simulink model "hybrid_5_bus_scan_comparison"  (R2024b)
settings: Solver=FixedStepAuto  StartTime=0  StopTime=200  FixedStep=Ts  RelTol=1e-3
PreLoadFcn:
  | Ts = 1e-5;FS_Frequency=csvread('Frequency_Sweep.csv',1,0); run lpf_param.m;
InitFcn:
  | Ts = 1e-5;FS_Frequency=csvread('Frequency_Sweep.csv',1,0); run lpf_param.m;
StartFcn:
  | Ts = 1e-5;FS_Frequency=csvread('Frequency_Sweep.csv',1,0); run lpf_param.m;
values from neighbouring files (symbols this model uses):
  D = zeros(6,4)    [TheoreticalImpedancePlot.m]    (also in TheoreticalImpedancePlotGFL.m = zeros(5,4))
  Fbase = 50    [lpf_param.m]
  fpll = 0.1    [lpf_param.m]
  k_lpf = 0.707    [lpf_param.m]
  wc_lpf = 2*pi*fc_lpf    (= 0.628318530718)    [lpf_param.m]
  x_e = [i_d; i_q; i_d_i; i_q_i; v_d_i; v_q_i; theta; v_dc; v_dc_i; i; i_i; v_lk; p_sum_i; p_lk_i]    [InterlinkAcDcB2B.m]
undefined symbols (not defined in the file or in its folder): ApparatusDiscreDamping, ApparatusPara, ApparatusPowerFlow, ApparatusType, DiscIntNeverNeededParam, OtherInputs, Wbase, Ybase, Zbase
libraries: SimplusGT x20, discretizing x12, dspindex x8, spsGroundLib x5, dspsnks4 x4, spsThreePhaseParallelRLCBranchLib x3, spsControlledVoltageSourceLib x3, spsThreePhaseSeriesRLCBranchLib x2, spsParallelRLCBranchLib x2, spsThreePhaseVIMeasurementLib x2, simulink x1, sps_lib x1
(part 1 of 2)
settings Model: Creator=gzhan  LastModifiedBy=gzhan

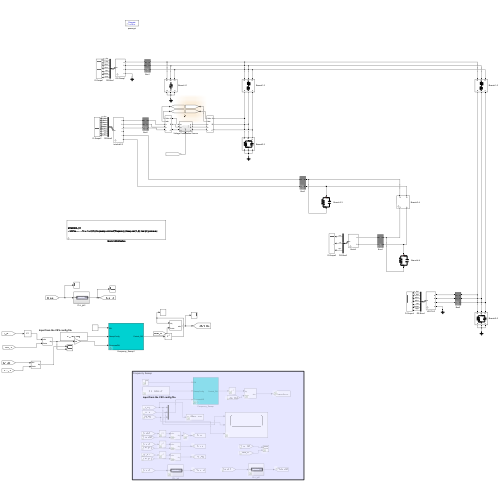
[thumbnail: Simulink's stored preview of the top-level diagram]
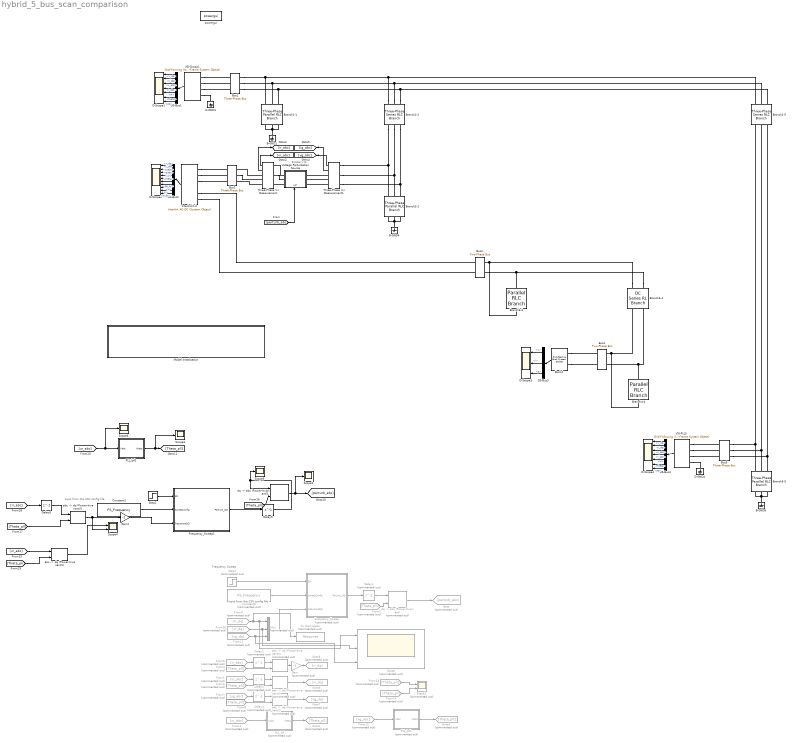
== system hybrid_5_bus_scan_comparison ==
  note: $\tilde{v}$
  note: Input from the CSV config file.
  note: Frequency Sweep
  note: Input from the CSV config file.
  B-GND1 : spsGroundLib/Ground  LConnTagsString=a
  B-GND4 : spsGroundLib/Ground  LConnTagsString=a
  B-GND8 : spsGroundLib/Ground  LConnTagsString=a
  Branch1-1 : spsThreePhaseParallelRLCBranchLib/Three-Phase Parallel RLC Branch  LConnTagsString=A|B|C  RConnTagsString=A|B|C  BranchType=C  Resistance=(Inf)*Zbase  Inductance=(Inf)*Zbase/Wbase  Capacitance=(0.0001)*Ybase/Wbase  Measurements=None
  Branch1-2 : spsThreePhaseSeriesRLCBranchLib/Three-Phase Series RLC Branch  LConnTagsString=A|B|C  RConnTagsString=A|B|C  BranchType=RL  Resistance=(0.01)*Zbase  Inductance=(0.3)*Zbase/Wbase  Capacitance=1e-6  Measurements=None
  Branch1-5 : spsThreePhaseSeriesRLCBranchLib/Three-Phase Series RLC Branch  LConnTagsString=A|B|C  RConnTagsString=A|B|C  BranchType=RL  Resistance=(0.01)*Zbase  Inductance=(0.3)*Zbase/Wbase  Capacitance=1e-6  Measurements=None
  Branch2-2 : spsThreePhaseParallelRLCBranchLib/Three-Phase Parallel RLC Branch  LConnTagsString=A|B|C  RConnTagsString=A|B|C  BranchType=RC  Resistance=(1.7547)*Zbase  Inductance=(Inf)*Zbase/Wbase  Capacitance=(0.0001)*Ybase/Wbase  Measurements=None
  Branch3-3 : spsParallelRLCBranchLib/Parallel RLC Branch  LConnTagsString=a  RConnTagsString=__new0  BranchType=RC  Resistance=(2)*Zbase  Inductance=(Inf)*Zbase/Wbase  SetiL0=off  InitialCurrent=0  Capacitance=(0.0001)*Ybase/Wbase  Setx0=off  InitialVoltage=0  Measurements=None
  Branch3-4 : SimplusGT/DC Series RL Branch  BranchType=RL  Resistance=(0.01)*Zbase  Inductance=(0.3)*Zbase/Wbase
      settings: SourceProductName=Simplus Grid Tool
  Branch4-4 : spsParallelRLCBranchLib/Parallel RLC Branch  LConnTagsString=a  RConnTagsString=__new0  BranchType=RC  Resistance=(2)*Zbase  Inductance=(Inf)*Zbase/Wbase  SetiL0=off  InitialCurrent=0  Capacitance=(0.0001)*Ybase/Wbase  Setx0=off  InitialVoltage=0  Measurements=None
  Branch5-5 : spsThreePhaseParallelRLCBranchLib/Three-Phase Parallel RLC Branch  LConnTagsString=A|B|C  RConnTagsString=A|B|C  BranchType=RC  Resistance=(2.0009)*Zbase  Inductance=(Inf)*Zbase/Wbase  Capacitance=(0.0001)*Ybase/Wbase  Measurements=None
  Buck4 : SimplusGT/Grid-Feeding Buck (System Object)  Ts=Ts  Sbase=Sbase  Vbase=Vbase  ApparatusType=ApparatusType{3}  ApparatusPara=ApparatusPara{3}  PowerFlow=ApparatusPowerFlow{3}  x0=x_e{3}  OtherInputs=OtherInputs{3}  DiscreMethod=Hybrid Trapezoidal  EnableInsideModification=off  DiscreDampingFlag=on  DiscreDampingValue=ApparatusDiscreDamping{3}  LinearizationTimes=1  DirectFeedthrough=off
      settings: SourceProductName=Simplus Grid Tool
  Bus1 : SimplusGT/Three-Phase Bus  Vbase=1  Sbase=1
      settings: SourceProductName=Simplus Grid Tool
  Bus2 : SimplusGT/Three-Phase Bus  Vbase=1  Sbase=1
      settings: SourceProductName=Simplus Grid Tool
  Bus3 : SimplusGT/Two-Phase Bus  Vbase=1  Sbase=1
      settings: SourceProductName=Simplus Grid Tool
  Bus4 : SimplusGT/Two-Phase Bus  Vbase=1  Sbase=1
      settings: SourceProductName=Simplus Grid Tool
  Bus5 : SimplusGT/Three-Phase Bus  Vbase=1  Sbase=1
      settings: SourceProductName=Simplus Grid Tool
  Constant1 : Constant  Value=FS_Frequency
  Constant8 : Constant  Commented=on  Value=FS_Frequency
  D-GND1 : spsGroundLib/Ground  LConnTagsString=a
  D-GND4 : spsGroundLib/Ground  LConnTagsString=a
  D-Scope1 : Scope  NumInputPorts=7
  D-Scope2 : Scope  NumInputPorts=10
  D-Scope3 : Scope  NumInputPorts=3
  D-Scope4 : Scope  NumInputPorts=7
  DS-Bus1 : BusSelector  OutputSignals=v_dq,i_dq,v_abc,i_abc,w,theta,pq
  DS-Bus2 : BusSelector  OutputSignals=v_dq,i_dq,v_abc,i_abc,w,theta,pq_ac,v,i,p_dc
  DS-Bus3 : BusSelector  OutputSignals=v,i,p
  DS-Bus4 : BusSelector  OutputSignals=v_dq,i_dq,v_abc,i_abc,w,theta,pq
  Delay{1..4} (4 alike) : Delay  Commented=on  DelayLength=1
  Delay5 : Delay  DelayLength=1
  Delay6 : Delay  DelayLength=1
  Frequency_Sweep : Subsystem  Commented=on  mask{Gain=0.02, Interval=1e-2}
      mask prompts: Gain "Output Gain"; Interval "Injection Interval"
  Frequency_Sweep1 : Subsystem  mask{Gain=0.02, Interval=1e-2}
      mask prompts: Gain "Output Gain"; Interval "Injection Interval"
  From1 : From  Commented=on  GotoTag=vr_abc
  From10 : From  Commented=on  GotoTag=vr_dq
  From11 : From  Commented=on  GotoTag=vg_dq
  From12 : From  Commented=on  GotoTag=vg_abc
  From{2,4,6,8,13} (5 alike) : From  Commented=on  GotoTag=Theta_pll2
  From14 : From  Commented=on  GotoTag=Theta_pll
  From3 : From  Commented=on  GotoTag=vr_abc
  From5 : From  Commented=on  GotoTag=ir_abc
  From7 : From  Commented=on  GotoTag=vg_abc
  From9 : From  Commented=on  GotoTag=ir_dq
  Gain : Gain  Commented=on  Gain=-1
  Gain1 : Gain  Gain=-1
  Goto : Goto  Commented=on  GotoTag=perturb_abc
  Goto1 : Goto  Commented=on  GotoTag=Theta_pll
  Goto6 : Goto  Commented=on  GotoTag=vr_dq
  Goto7 : Goto  Commented=on  GotoTag=vg_dq
  Goto8 : Goto  Commented=on  GotoTag=ir_dq
  Goto9 : Goto  Commented=on  GotoTag=Theta_pll2
  Interlink2-3 : SimplusGT/Interlink AC-DC (System Object)  Ts=Ts  Sbase=Sbase  Vbase=Vbase  Wbase=Wbase  ApparatusType=ApparatusType{2}  ApparatusPara=ApparatusPara{2}  PowerFlow=ApparatusPowerFlow{2}  x0=x_e{2}  OtherInputs=OtherInputs{2}  DiscreMethod=Hybrid Trapezoidal  EnableInsideModification=off  DiscreDampingFlag=on  DiscreDampingValue=ApparatusDiscreDamping{2}  LinearizationTimes=1  DirectFeedthrough=off
      settings: SourceProductName=Simplus Grid Tool
  Model Initialization : Subsystem  mask(Model Functions){InitFcnVar=Ts = 1e-5;FS_Frequency=csvread('Frequency_Sweep.csv',1,0); run lpf_param.m;}
      mask prompts: InitFcnVar "InitFcn"
      mask init:
      | set_param(bdroot, 'PreLoadFcn', InitFcnVar);
      | set_param(bdroot, 'InitFcn', InitFcnVar);
      | set_param(bdroot, 'StartFcn', InitFcnVar);
      | PLF = get_param(bdroot, 'PreLoadFcn');
      | IF = get_param(bdroot, 'InitFcn');
      | SF = get_param(bdroot, 'StartFcn');
      | 
      | 
      | pos = get_param(gcb, 'Position');
      | width = pos(3) - pos(1); height = pos(4) - pos(2);
      mask Display:
      | text(5, height*0.5, [ ...
      | upper(bdroot) '\n' ...
      | '- InitFcn. . . . . '  get_param(bdroot, 'InitFcn')  ...
      | ], ...
      | 'horizontalAlignment', 'left', 'verticalAlignment', 'middle') ;
  Mux : Mux  Commented=on  Inputs=3
  PLL_lpf : Subsystem  Commented=on
  PLL_lpf1 : Subsystem  Commented=on
  PLL_lpf2 : Subsystem
  Scope : Scope  Commented=on  NumInputPorts=3
  Scope1 : Scope  Commented=on  NumInputPorts=2
  Scope{2..3,5..6} (4 alike) : Scope
  Scope4 : Scope  NumInputPorts=2
  Step1 : Step  Commented=on  Time=4  SampleTime=0
  Step2 : Step  Time=4  SampleTime=0
  Three-Phase V-I Measurement : spsThreePhaseVIMeasurementLib/Three-Phase V-I Measurement  VoltageMeasurement=phase-to-ground  SetLabelV=off  LabelV=Vabc_mea  Vpu=off  VpuLL=off  CurrentMeasurement=yes  SetLabelI=off  LabelI=Iabc_mea  Ipu=off  Pbase=100e6  Vbase=500e3  OutputType=Complex  PhasorSimulation=off  PSBequivalent=0
  Three-Phase V-I Measurement1 : spsThreePhaseVIMeasurementLib/Three-Phase V-I Measurement  VoltageMeasurement=phase-to-ground  SetLabelV=off  LabelV=Vabc_mea  Vpu=off  VpuLL=off  CurrentMeasurement=yes  SetLabelI=off  LabelI=Iabc_mea  Ipu=off  Pbase=100e6  Vbase=500e3  OutputType=Complex  PhasorSimulation=off  PSBequivalent=0
  To Workspace : ToWorkspace  Commented=on  VariableName=Response  SampleTime=-1
  VSI-Droop1 : SimplusGT/Grid-Forming Voltage-Source Inverter (dq-Frame System Object)  Ts=Ts  Sbase=Sbase  Vbase=Vbase  Wbase=Wbase  ApparatusType=ApparatusType{1}  ApparatusPara=ApparatusPara{1}  PowerFlow=ApparatusPowerFlow{1}  x0=x_e{1}  OtherInputs=OtherInputs{1}  DiscreMethod=Hybrid Trapezoidal  EnableInsideModification=off  DiscreDampingFlag=on  DiscreDampingValue=ApparatusDiscreDamping{1}  LinearizationTimes=1  DirectFeedthrough=off
      settings: SourceProductName=Simplus Grid Tool
  VSI-PLL5 : SimplusGT/Grid-Following Voltage-Source Inverter (dq-Frame System Object)  Ts=Ts  Sbase=Sbase  Vbase=Vbase  Wbase=Wbase  ApparatusType=ApparatusType{4}  ApparatusPara=ApparatusPara{4}  PowerFlow=ApparatusPowerFlow{4}  x0=x_e{4}  OtherInputs=OtherInputs{4}  DiscreMethod=Hybrid Trapezoidal  EnableInsideModification=off  DiscreDampingFlag=on  DiscreDampingValue=ApparatusDiscreDamping{4}  LinearizationTimes=1  DirectFeedthrough=off
      settings: SourceProductName=Simplus Grid Tool
  Voltage Perturbation Source : Subsystem
      settings: PortSchema="{\"entries\":[{\"content\":{\"sides\":[{\"content\":{\"connectorIds\":[\"LConn1\",\"LConn2\",\"LConn3\"]},\"type\":\"ConnectorPlacement.EquallySpacedRectSide\",\"uuid\":\"6f603e87-6b2e-4585-ad3a-55936445c397\"},{\"content\":{\"connectorIds\":[\"RConn1\",\"RConn2\",\"RConn3\"],\"side\":\"RIGHT\"},\"type\":\"ConnectorPlacement.EquallySpacedRectSide\",\"uuid\":\"08c5aebc-ed45-455a-9198-e657d358a757\"},{\"content\":{\"side\":\"TOP\"},\"type\":\"ConnectorPlacement.EquallySpacedRectSide\",\"uuid\":\"90e892ab-d7d1-4f2e-b125-0b742fd1657c\"},{\"content\":{\"connectorIds\":[\"In1\"],\"side\":\"BOTTOM\"},\"type\":\"ConnectorPlacement.EquallySpacedRectSide\",\"uuid\":\"ba12d237-2ee0-4e5a-b3d4-1de3f90cbef1\"}]},\"type\":\"ConnectorPlacement.EquallySpacedConnector\",\"uuid\":\"0150c08c-ed05-4e99-aa85-f9e708dbbe93\"}],\"packageUris\":[\"http://schema.mathworks.com/mf0/Connector/R2020b\"],\"version\":\"1.0\"}"
  "abc -> dq (Power-Invariant)1" : SimplusGT/abc -> dq (Power-Invariant)  Commented=on  SystemSampleTime=-1  VariantActivationTime=update diagram  AllowFlexibleInterface=on  Latency=0  AutoFrameSizeCalculation=off
      settings: SourceProductName=Simplus Grid Tool
  "abc -> dq (Power-Invariant)2" : SimplusGT/abc -> dq (Power-Invariant)  Commented=on  SystemSampleTime=-1  VariantActivationTime=update diagram  AllowFlexibleInterface=on  Latency=0  AutoFrameSizeCalculation=off
      settings: SourceProductName=Simplus Grid Tool
  "abc -> dq (Power-Invariant)3" : SimplusGT/abc -> dq (Power-Invariant)  SystemSampleTime=-1  VariantActivationTime=update diagram  AllowFlexibleInterface=on  Latency=0  AutoFrameSizeCalculation=off
      settings: SourceProductName=Simplus Grid Tool
  "abc -> dq (Power-Invariant)4" : SimplusGT/abc -> dq (Power-Invariant)  Commented=on  SystemSampleTime=-1  VariantActivationTime=update diagram  AllowFlexibleInterface=on  Latency=0  AutoFrameSizeCalculation=off
      settings: SourceProductName=Simplus Grid Tool
  "abc -> dq (Power-Invariant)5" : SimplusGT/abc -> dq (Power-Invariant)  SystemSampleTime=-1  VariantActivationTime=update diagram  AllowFlexibleInterface=on  Latency=0  AutoFrameSizeCalculation=off
      settings: SourceProductName=Simplus Grid Tool
  "dq -> abc (Power-Invariant)" : SimplusGT/dq -> abc (Power-Invariant)  Commented=on  SystemSampleTime=-1  VariantActivationTime=update diagram  AllowFlexibleInterface=on  Latency=0  AutoFrameSizeCalculation=off
      settings: SourceProductName=Simplus Grid Tool
  "dq -> abc (Power-Invariant)1" : SimplusGT/dq -> abc (Power-Invariant)  SystemSampleTime=-1  VariantActivationTime=update diagram  AllowFlexibleInterface=on  Latency=0  AutoFrameSizeCalculation=off
      settings: SourceProductName=Simplus Grid Tool
  powergui : sps_lib/powergui  Priority=1  SimulationMode=Discrete  SampleTime=Ts  frequency=60  Iterations=50  frequencyindice=0  Pbase=100e6  ErrMax=1e-4  UnitsV=kV  UnitsW=MW  buscounter=0  FunctionMessages=off  echomessages=off  EnableUseOfTLC=off  CurrentSourceSwitches=off  DisableSnubberDevices=off  DisableRonSwitches=off  DisableVfSwitches=off  DisplayEquations=off  AutomaticDiscreteSolvers=off  SolverType=Tustin/Backward Euler (TBE)  Interpol=off  ExternalGateDelay=off  methode=off  Ts=100  x0status=blocks  SPID=on  SwTol=0  HookPort=off  NonlinearTolerance=1e-4  nMaxIteration=100  ContinueOnMaxIteration=off  RestoreLinks=warning  ResistiveCurrentMeasurement=off  Frange=[0:2:500]  Ylog=off  Xlog=on  ShowGrid=off  save=off  variable=ZData  structure=0  ZoomFFT=off  StartTime=0.0  cycles=1  DisplayStyle=1  fundamental=60  FreqAxis=off  MaxFrequency=1000  frequencyindicesteady=1  RmsSteady=1  display=off
  wires:
  VSI-Droop1/1 -> DS-Bus1/1
  DS-Bus1/1 -> D-Scope1/1  "<v_dq>"
  DS-Bus1/2 -> D-Scope1/2  "<i_dq>"
  DS-Bus1/3 -> D-Scope1/3  "<v_abc>"
  DS-Bus1/4 -> D-Scope1/4  "<i_abc>"
  DS-Bus1/5 -> D-Scope1/5  "<w>"
  DS-Bus1/6 -> D-Scope1/6  "<theta>"
  DS-Bus1/7 -> D-Scope1/7  "<pq>"
  Interlink2-3/1 -> DS-Bus2/1
  DS-Bus2/1 -> D-Scope2/1  "<v_dq>"
  DS-Bus2/2 -> D-Scope2/2  "<i_dq>"
  DS-Bus2/3 -> D-Scope2/3  "<v_abc>"
  DS-Bus2/4 -> D-Scope2/4  "<i_abc>"
  DS-Bus2/5 -> D-Scope2/5  "<w>"
  DS-Bus2/6 -> D-Scope2/6  "<theta>"
  DS-Bus2/7 -> D-Scope2/7  "<pq_ac>"
  DS-Bus2/8 -> D-Scope2/8  "<v>"
  DS-Bus2/9 -> D-Scope2/9  "<i>"
  DS-Bus2/10 -> D-Scope2/10  "<p_dc>"
  Buck4/1 -> DS-Bus3/1
  DS-Bus3/1 -> D-Scope3/1  "<v>"
  DS-Bus3/2 -> D-Scope3/2  "<i>"
  DS-Bus3/3 -> D-Scope3/3  "<p>"
  VSI-PLL5/1 -> DS-Bus4/1
  DS-Bus4/1 -> D-Scope4/1  "<v_dq>"
  DS-Bus4/2 -> D-Scope4/2  "<i_dq>"
  DS-Bus4/3 -> D-Scope4/3  "<v_abc>"
  DS-Bus4/4 -> D-Scope4/4  "<i_abc>"
  DS-Bus4/5 -> D-Scope4/5  "<w>"
  DS-Bus4/6 -> D-Scope4/6  "<theta>"
  DS-Bus4/7 -> D-Scope4/7  "<pq>"
  Three-Phase V-I Measurement1/1 -> [vg_abc]
  Three-Phase V-I Measurement1/2 -> [ig_abc]
  Three-Phase V-I Measurement/2 -> [ir_abc]
  Three-Phase V-I Measurement/1 -> [vr_abc]
  [perturb_abc] -> Voltage Perturbation Source/1(ref)
  From14/1 -> Scope1/2
  From1/1 -> Delay3/1
  Delay2/1 -> "abc -> dq (Power-Invariant)4"/1
  "abc -> dq (Power-Invariant)2"/1 -> Goto7/1
  Step1/1 -> Frequency_Sweep/1(EN)
  "dq -> abc (Power-Invariant)"/1 -> Goto/1
  From2/1 -> "dq -> abc (Power-Invariant)"/2
  From10/1 -> Scope/2, Mux/2
  From6/1 -> "abc -> dq (Power-Invariant)1"/2
  Constant8/1 -> Frequency_Sweep/2(SweepConfig)
  From12/1 -> PLL_lpf1/1(Vabc)
  From7/1 -> Delay4/1
  From13/1 -> Scope1/1
  Gain/1 -> Goto8/1
  From8/1 -> "abc -> dq (Power-Invariant)2"/2
  Delay1/1 -> "dq -> abc (Power-Invariant)"/1
  From5/1 -> Delay2/1
  "abc -> dq (Power-Invariant)1"/1 -> Goto6/1
  Delay4/1 -> "abc -> dq (Power-Invariant)2"/1
  From9/1 -> To Workspace/1, Scope/1, Mux/1
  PLL_lpf/1(theta) -> Goto1/1
  Delay3/1 -> "abc -> dq (Power-Invariant)1"/1
  From3/1 -> PLL_lpf/1(Vabc)
  PLL_lpf1/1(theta) -> Goto9/1
  From11/1 -> Scope/3, Mux/3
  Frequency_Sweep/1(Perturb_DQ) -> Delay1/1
  "abc -> dq (Power-Invariant)4"/1 -> Gain/1
  Mux/1 -> Frequency_Sweep/3(ResponseDQ)
  From4/1 -> "abc -> dq (Power-Invariant)4"/2
  [Theta_pll] -> "abc -> dq (Power-Invariant)3"/2
  Step2/1 -> Frequency_Sweep1/1(EN)
  "abc -> dq (Power-Invariant)3"/1 -> Scope4/1
  [Theta_pll] -> "dq -> abc (Power-Invariant)1"/2
  Constant1/1 -> Frequency_Sweep1/2(SweepConfig)
  "abc -> dq (Power-Invariant)5"/1 -> Scope4/2, Gain1/1
  [ir_abc] -> Delay6/1
  [Theta_pll] -> "abc -> dq (Power-Invariant)5"/2
  Delay6/1 -> "abc -> dq (Power-Invariant)5"/1
  Delay5/1 -> "dq -> abc (Power-Invariant)1"/1, Scope5/1
  Gain1/1 -> Frequency_Sweep1/3(ResponseDQ)
  Frequency_Sweep1/1(Perturb_DQ) -> Delay5/1
  "dq -> abc (Power-Invariant)1"/1 -> Scope2/1, [perturb_abc]
  [vr_abc] -> "abc -> dq (Power-Invariant)3"/1
  [vr_abc] -> Scope6/1, PLL_lpf2/1(Vabc)
  PLL_lpf2/1(theta) -> Scope3/1, [Theta_pll]
  connections:
  VSI-Droop1/LConn4 -- D-GND1/LConn1
  VSI-PLL5/LConn4 -- D-GND4/LConn1
  Branch1-1/RConn1 -- Branch1-1/RConn2 -- Branch1-1/RConn3 -- B-GND1/LConn1
  Branch2-2/RConn1 -- Branch2-2/RConn2 -- Branch2-2/RConn3 -- B-GND4/LConn1
  Branch5-5/RConn1 -- Branch5-5/RConn2 -- Branch5-5/RConn3 -- B-GND8/LConn1
  Branch1-2/RConn1 -- Three-Phase V-I Measurement1/LConn1 -- Branch2-2/LConn1
  Branch1-2/RConn2 -- Three-Phase V-I Measurement1/LConn2 -- Branch2-2/LConn2
  Branch1-2/RConn3 -- Three-Phase V-I Measurement1/LConn3 -- Branch2-2/LConn3
  Branch1-2/LConn1 -- Bus1/RConn1 -- Branch1-1/LConn1 -- Branch1-5/LConn1
  Branch1-2/LConn2 -- Bus1/RConn2 -- Branch1-1/LConn2 -- Branch1-5/LConn2
  Branch1-2/LConn3 -- Bus1/RConn3 -- Branch1-1/LConn3 -- Branch1-5/LConn3
  Branch1-5/RConn1 -- Bus5/RConn1 -- Branch5-5/LConn1
  Branch1-5/RConn2 -- Bus5/RConn2 -- Branch5-5/LConn2
  Branch1-5/RConn3 -- Bus5/RConn3 -- Branch5-5/LConn3
  Branch3-4/RConn1 -- Bus4/RConn1 -- Branch4-4/RConn1
  Branch3-4/RConn2 -- Bus4/RConn2 -- Branch4-4/LConn1
  Branch3-4/LConn1 -- Bus3/RConn1 -- Branch3-3/RConn1
  Branch3-4/LConn2 -- Bus3/RConn2 -- Branch3-3/LConn1
  VSI-Droop1/LConn1 -- Bus1/LConn1
  VSI-Droop1/LConn2 -- Bus1/LConn2
  VSI-Droop1/LConn3 -- Bus1/LConn3
  Interlink2-3/LConn1 -- Bus2/LConn1
  Interlink2-3/LConn2 -- Bus2/LConn2
  Interlink2-3/LConn3 -- Bus2/LConn3
  Interlink2-3/LConn5 -- Bus3/LConn1
  Interlink2-3/LConn6 -- Bus3/LConn2
  Buck4/LConn1 -- Bus4/LConn1
  Buck4/LConn2 -- Bus4/LConn2
  VSI-PLL5/LConn1 -- Bus5/LConn1
  VSI-PLL5/LConn2 -- Bus5/LConn2
  VSI-PLL5/LConn3 -- Bus5/LConn3
  Voltage Perturbation Source/RConn1 -- Three-Phase V-I Measurement/LConn1
  Three-Phase V-I Measurement1/RConn3 -- Voltage Perturbation Source/LConn3
  Three-Phase V-I Measurement1/RConn1 -- Voltage Perturbation Source/LConn1
  Three-Phase V-I Measurement/LConn2 -- Voltage Perturbation Source/RConn2
  Voltage Perturbation Source/RConn3 -- Three-Phase V-I Measurement/LConn3
  Three-Phase V-I Measurement1/RConn2 -- Voltage Perturbation Source/LConn2
  Three-Phase V-I Measurement/RConn1 -- Bus2/RConn1
  Bus2/RConn2 -- Three-Phase V-I Measurement/RConn2
  Three-Phase V-I Measurement/RConn3 -- Bus2/RConn3

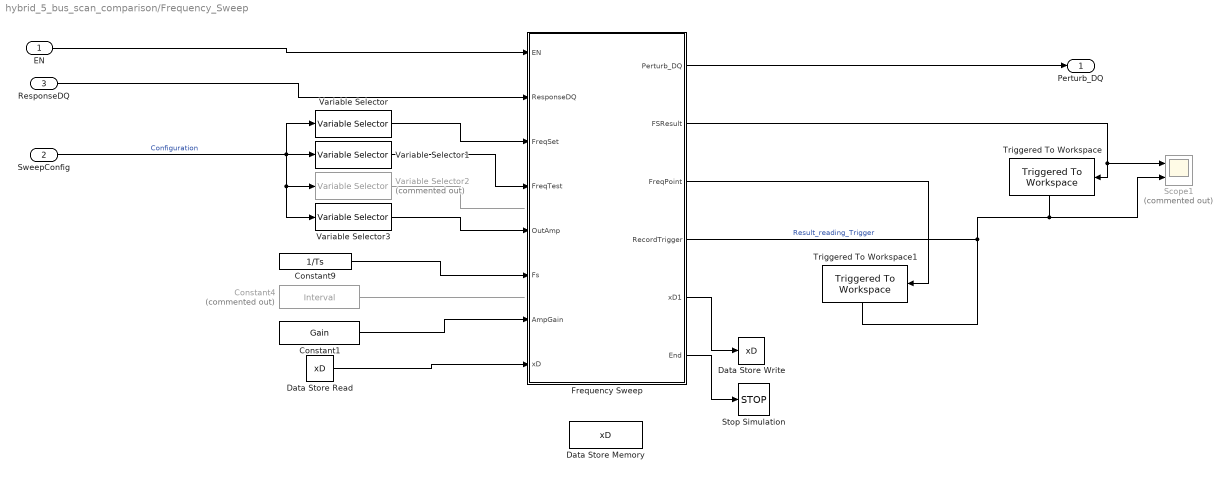
== system hybrid_5_bus_scan_comparison/Frequency_Sweep ==
  EN : Inport
  SweepConfig : Inport  Port=2
  ResponseDQ : Inport  Port=3
  Constant1 : Constant  Value=Gain
  Constant4 : Constant  Commented=on  Value=Interval
  Constant9 : Constant  Value=1/Ts
  Data Store Memory : DataStoreMemory  DataStoreName=xD  WriteAfterWriteMsg=warning  InitialValue=zeros(57,1)  ShowAdditionalParam=off
  Data Store Read : DataStoreRead  DataStoreName=xD  IndexOptions=Index vector (dialog)  Indices=1  OutputSizes=1
  Data Store Write : DataStoreWrite  DataStoreName=xD  IndexOptions=Index vector (dialog)  Indices=1  OutputSizes=1
  Frequency Sweep : MATLAB Function  TreatAsAtomicUnit=on
  Scope1 : Scope  Commented=on  NumInputPorts=2
  Stop Simulation : Stop
  Triggered To Workspace : dspsnks4/Triggered To Workspace  TriggerType=Rising edge  VariableName=FS_Result  Buffer=5000  Save2DMode=2-D array (concatenate along first dimension)
      settings: FixptAsFi=off
  Triggered To Workspace1 : dspsnks4/Triggered To Workspace  TriggerType=Rising edge  VariableName=FS_Freq_point  Buffer=5000  Save2DMode=2-D array (concatenate along first dimension)
      settings: FixptAsFi=off
  Variable Selector : dspindex/Variable Selector  NumInputs=1  rowsOrCols=Columns  IdxMode=Fixed  Elements=1  ZerOneIdxMode=One-based  errmode=Clip Index  FillMode=on  FillValues=0
  Variable Selector1 : dspindex/Variable Selector  NumInputs=1  rowsOrCols=Columns  IdxMode=Fixed  Elements=2  ZerOneIdxMode=One-based  errmode=Clip Index  FillMode=on  FillValues=0
  Variable Selector2 : dspindex/Variable Selector  Commented=on  NumInputs=1  rowsOrCols=Columns  IdxMode=Fixed  Elements=3  ZerOneIdxMode=One-based  errmode=Clip Index  FillMode=on  FillValues=0
  Variable Selector3 : dspindex/Variable Selector  NumInputs=1  rowsOrCols=Columns  IdxMode=Fixed  Elements=4  ZerOneIdxMode=One-based  errmode=Clip Index  FillMode=on  FillValues=0
  Perturb_DQ : Outport
  wires:
  Variable Selector2/1 -> ?
  Frequency Sweep/2(FSResult) -> Triggered To Workspace/1, Scope1/1
  Frequency Sweep/4(RecordTrigger) -> Triggered To Workspace1/Trigger, Scope1/2, Triggered To Workspace/Trigger  "Result_reading_Trigger"
  Constant4/1 -> ?
  Frequency Sweep/5(xD1) -> Data Store Write/1
  Variable Selector3/1 -> Frequency Sweep/5(OutAmp)
  Variable Selector1/1 -> Frequency Sweep/4(FreqTest)
  SweepConfig/1 -> Variable Selector3/1, Variable Selector2/1, Variable Selector1/1, Variable Selector/1  "Configuration"
  ResponseDQ/1 -> Frequency Sweep/2(ResponseDQ)
  Variable Selector/1 -> Frequency Sweep/3(FreqSet)
  Frequency Sweep/3(FreqPoint) -> Triggered To Workspace1/1
  Data Store Read/1 -> Frequency Sweep/8(xD)
  Constant9/1 -> Frequency Sweep/6(Fs)
  Frequency Sweep/1(Perturb_DQ) -> Perturb_DQ/1
  EN/1 -> Frequency Sweep/1(EN)
  Constant1/1 -> Frequency Sweep/7(AmpGain)
  Frequency Sweep/6(End) -> Stop Simulation/1

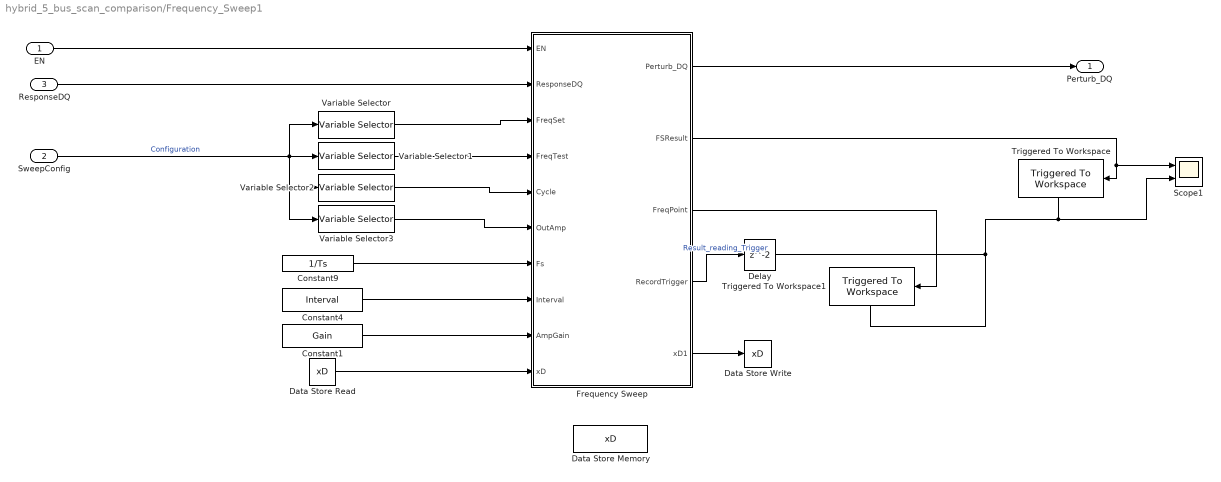
== system hybrid_5_bus_scan_comparison/Frequency_Sweep1 ==
  EN : Inport
  SweepConfig : Inport  Port=2
  ResponseDQ : Inport  Port=3
  Constant1 : Constant  Value=Gain
  Constant4 : Constant  Value=Interval
  Constant9 : Constant  Value=1/Ts
  Data Store Memory : DataStoreMemory  DataStoreName=xD  WriteAfterWriteMsg=warning  InitialValue=zeros(1,16)  ShowAdditionalParam=off
  Data Store Read : DataStoreRead  DataStoreName=xD  IndexOptions=Index vector (dialog)  Indices=1  OutputSizes=1
  Data Store Write : DataStoreWrite  DataStoreName=xD  IndexOptions=Index vector (dialog)  Indices=1  OutputSizes=1
  Delay : Delay
  Frequency Sweep : MATLAB Function  TreatAsAtomicUnit=on
  Scope1 : Scope  NumInputPorts=2
  Triggered To Workspace : dspsnks4/Triggered To Workspace  TriggerType=Rising edge  VariableName=FS_Result  Buffer=5000  Save2DMode=2-D array (concatenate along first dimension)
      settings: FixptAsFi=off
  Triggered To Workspace1 : dspsnks4/Triggered To Workspace  TriggerType=Rising edge  VariableName=FS_Freq_point  Buffer=5000  Save2DMode=2-D array (concatenate along first dimension)
      settings: FixptAsFi=off
  Variable Selector : dspindex/Variable Selector  NumInputs=1  rowsOrCols=Columns  IdxMode=Fixed  Elements=1  ZerOneIdxMode=One-based  errmode=Clip Index  FillMode=on  FillValues=0
  Variable Selector1 : dspindex/Variable Selector  NumInputs=1  rowsOrCols=Columns  IdxMode=Fixed  Elements=2  ZerOneIdxMode=One-based  errmode=Clip Index  FillMode=on  FillValues=0
  Variable Selector2 : dspindex/Variable Selector  NumInputs=1  rowsOrCols=Columns  IdxMode=Fixed  Elements=3  ZerOneIdxMode=One-based  errmode=Clip Index  FillMode=on  FillValues=0
  Variable Selector3 : dspindex/Variable Selector  NumInputs=1  rowsOrCols=Columns  IdxMode=Fixed  Elements=4  ZerOneIdxMode=One-based  errmode=Clip Index  FillMode=on  FillValues=0
  Perturb_DQ : Outport
  wires:
  Variable Selector2/1 -> Frequency Sweep/5(Cycle)
  Frequency Sweep/2(FSResult) -> Triggered To Workspace/1, Scope1/1
  Frequency Sweep/4(RecordTrigger) -> Delay/1  "Result_reading_Trigger"
  Constant4/1 -> Frequency Sweep/8(Interval)
  Frequency Sweep/5(xD1) -> Data Store Write/1
  Variable Selector3/1 -> Frequency Sweep/6(OutAmp)
  Variable Selector1/1 -> Frequency Sweep/4(FreqTest)
  SweepConfig/1 -> Variable Selector3/1, Variable Selector2/1, Variable Selector1/1, Variable Selector/1  "Configuration"
  ResponseDQ/1 -> Frequency Sweep/2(ResponseDQ)
  Variable Selector/1 -> Frequency Sweep/3(FreqSet)
  Frequency Sweep/3(FreqPoint) -> Triggered To Workspace1/1
  Data Store Read/1 -> Frequency Sweep/10(xD)
  Constant9/1 -> Frequency Sweep/7(Fs)
  Frequency Sweep/1(Perturb_DQ) -> Perturb_DQ/1
  EN/1 -> Frequency Sweep/1(EN)
  Delay/1 -> Scope1/2, Triggered To Workspace/Trigger, Triggered To Workspace1/Trigger
  Constant1/1 -> Frequency Sweep/9(AmpGain)

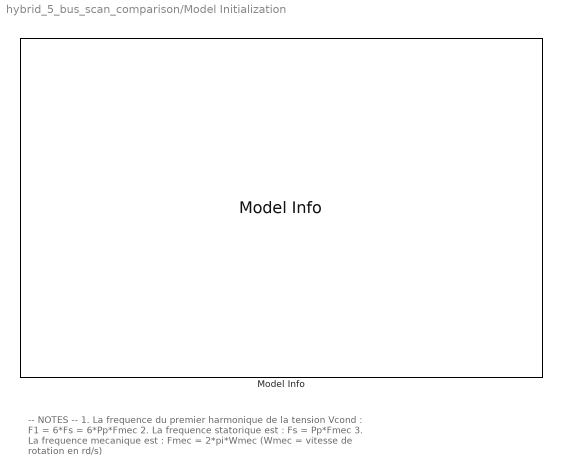
== system hybrid_5_bus_scan_comparison/Model Initialization ==
  note: -- NOTES --
      | 1. La frequence du premier harmonique de la tension Vcond :
      |     F1 = 6*Fs = 6*Pp*Fmec
      | 2. La frequence statorique est :
      |     Fs = Pp*Fmec
      | 3. La frequence mecanique est :
      |     Fmec = 2*pi*Wmec  (Wmec = vitesse de rotation en rd/s)
  Model Info : simulink/Model-Wide Utilities/Model Info  Frame=on  DisplayStringWithTags=|  HorizontalTextAlignment=Left  LeftAlignmentValue=0.02
      | - Version <<< %<ModelVersion> >>>
      | 
      | - Description :
      | %<Description>
      | 
      | - Created by :     %<Creator>
      | - Creation date : %<Created>
      | - Modified by :    %<ModifiedBy>
      | - Last modif. :     %<LastModificationDate>

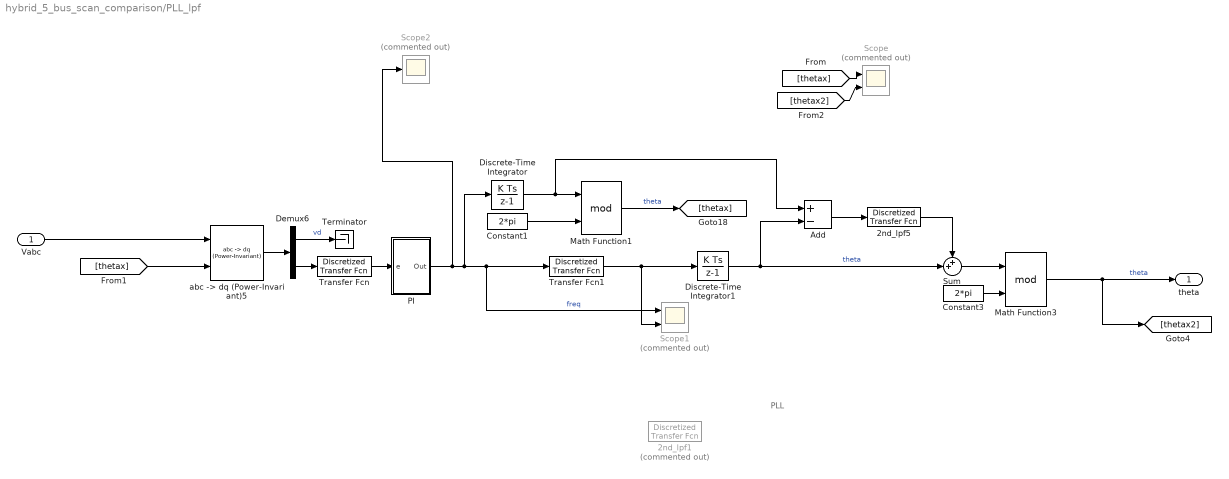
== system hybrid_5_bus_scan_comparison/PLL_lpf ==
  note: PLL
  Vabc : Inport
  2nd_lpf1 : discretizing/Discretized Transfer Fcn  Commented=on  Numerator=[wc_lpf^2]  Denominator="[1, 2*k_lpf*wc_lpf,  wc_lpf^2]"  AbsTol=auto  SampleTime=10e-6  method=zoh  Wc=0
  2nd_lpf5 : discretizing/Discretized Transfer Fcn  Numerator=[wc_lpf^2]  Denominator="[1, 2*k_lpf*wc_lpf,  wc_lpf^2]"  AbsTol=auto  SampleTime=Ts  method=zoh  Wc=0
  Add : Sum  Inputs=+-
  Constant1 : Constant  Value=2*pi
  Constant3 : Constant  Value=2*pi
  Demux6 : Demux  Outputs=2
  Discrete-Time Integrator : DiscreteIntegrator  SampleTime=Ts  ICPrevOutput=DiscIntNeverNeededParam  ICPrevScaledInput=DiscIntNeverNeededParam
  Discrete-Time Integrator1 : DiscreteIntegrator  SampleTime=Ts  ICPrevOutput=DiscIntNeverNeededParam  ICPrevScaledInput=DiscIntNeverNeededParam
  Math Function1 : Math  Operator=mod  SignedPower=on
  Math Function3 : Math  Operator=mod  SignedPower=on
  PI : Subsystem  mask{Kp_PLL=2*pi*fpll, Ki_PLL=(2*pi*fpll)^2/4, IntSat_PLL=20000}
      mask prompts: Kp_PLL "Proportional (P)"; Ki_PLL "Integral (I)"; IntSat_PLL "Integrator Saturation Limit"
      mask DialogControl DescGroupVar Prompt: PLL Parameters
  Scope : Scope  Commented=on  NumInputPorts=2
  Scope1 : Scope  Commented=on  NumInputPorts=2
  Scope2 : Scope  Commented=on
  Sum : Sum  Inputs=++|
  Terminator : Terminator
  Transfer Fcn : discretizing/Discretized Transfer Fcn  Numerator=[1]  Denominator=[1/(2*pi*50) 1]  AbsTol=auto  SampleTime=Ts  method=zoh  Wc=0
  Transfer Fcn1 : discretizing/Discretized Transfer Fcn  Numerator=[1]  Denominator=[1/(2*pi*1) 1]  AbsTol=auto  SampleTime=Ts  method=zoh  Wc=0
  "abc -> dq (Power-Invariant)5" : SimplusGT/abc -> dq (Power-Invariant)  SystemSampleTime=-1  VariantActivationTime=update diagram  AllowFlexibleInterface=on  Latency=0  AutoFrameSizeCalculation=off
      settings: SourceProductName=Simplus Grid Tool
  theta : Outport
  wires:
  Math Function3/1 -> theta/1, [thetax2]  "theta"
  Discrete-Time Integrator1/1 -> Sum/2, Add/2  "theta"
  Constant1/1 -> Math Function1/2
  Transfer Fcn/1 -> PI/1(e)
  Math Function1/1 -> [thetax]  "theta"
  Sum/1 -> Math Function3/1
  Transfer Fcn1/1 -> Scope1/2, Discrete-Time Integrator1/1
  Constant3/1 -> Math Function3/2
  [thetax] -> "abc -> dq (Power-Invariant)5"/2
  Demux6/2 -> Transfer Fcn/1
  PI/1(Out) -> Scope2/1, Transfer Fcn1/1, Scope1/1, Discrete-Time Integrator/1  "freq"
  "abc -> dq (Power-Invariant)5"/1 -> Demux6/1
  Add/1 -> 2nd_lpf5/1
  Demux6/1 -> Terminator/1  "vd"
  Vabc/1 -> "abc -> dq (Power-Invariant)5"/1
  Discrete-Time Integrator/1 -> Add/1, Math Function1/1
  [thetax] -> Scope/1
  [thetax2] -> Scope/2
  2nd_lpf5/1 -> Sum/1

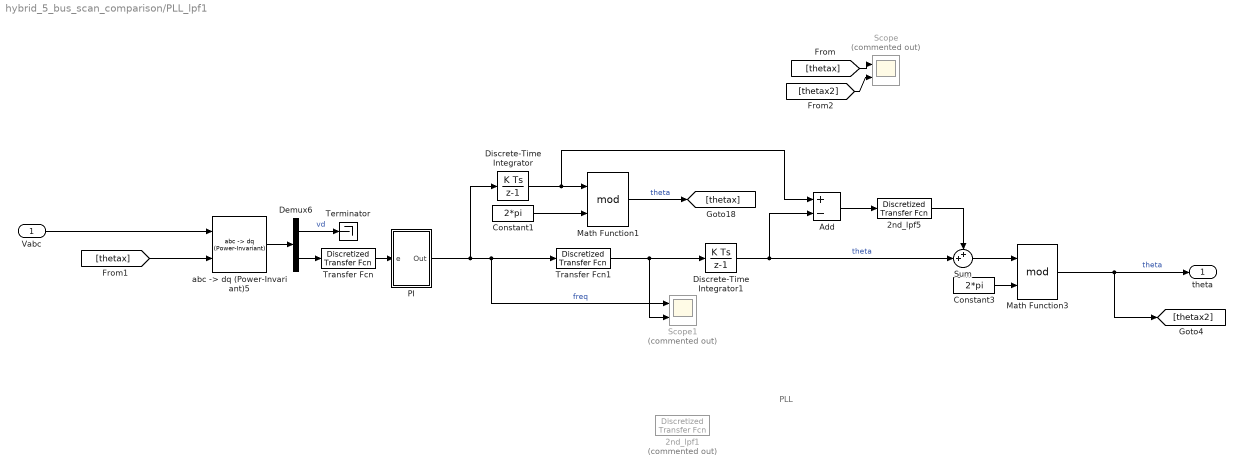
== system hybrid_5_bus_scan_comparison/PLL_lpf1 ==
  note: PLL
  Vabc : Inport
  2nd_lpf1 : discretizing/Discretized Transfer Fcn  Commented=on  Numerator=[wc_lpf^2]  Denominator="[1, 2*k_lpf*wc_lpf,  wc_lpf^2]"  AbsTol=auto  SampleTime=10e-6  method=zoh  Wc=0
  2nd_lpf5 : discretizing/Discretized Transfer Fcn  Numerator=[wc_lpf^2]  Denominator="[1, 2*k_lpf*wc_lpf,  wc_lpf^2]"  AbsTol=auto  SampleTime=Ts  method=zoh  Wc=0
  Add : Sum  Inputs=+-
  Constant1 : Constant  Value=2*pi
  Constant3 : Constant  Value=2*pi
  Demux6 : Demux  Outputs=2
  Discrete-Time Integrator : DiscreteIntegrator  SampleTime=Ts  ICPrevOutput=DiscIntNeverNeededParam  ICPrevScaledInput=DiscIntNeverNeededParam
  Discrete-Time Integrator1 : DiscreteIntegrator  SampleTime=Ts  ICPrevOutput=DiscIntNeverNeededParam  ICPrevScaledInput=DiscIntNeverNeededParam
  Math Function1 : Math  Operator=mod  SignedPower=on
  Math Function3 : Math  Operator=mod  SignedPower=on
  PI : Subsystem  mask{Kp_PLL=2*pi*fpll, Ki_PLL=(2*pi*fpll)^2/4, IntSat_PLL=20000}
      mask prompts: Kp_PLL "Proportional (P)"; Ki_PLL "Integral (I)"; IntSat_PLL "Integrator Saturation Limit"
      mask DialogControl DescGroupVar Prompt: PLL Parameters
  Scope : Scope  Commented=on  NumInputPorts=2
  Scope1 : Scope  Commented=on  NumInputPorts=2
  Sum : Sum  Inputs=++|
  Terminator : Terminator
  Transfer Fcn : discretizing/Discretized Transfer Fcn  Numerator=[1]  Denominator=[1/(2*pi*50) 1]  AbsTol=auto  SampleTime=Ts  method=zoh  Wc=0
  Transfer Fcn1 : discretizing/Discretized Transfer Fcn  Numerator=[1]  Denominator=[1/(2*pi*1) 1]  AbsTol=auto  SampleTime=Ts  method=zoh  Wc=0
  "abc -> dq (Power-Invariant)5" : SimplusGT/abc -> dq (Power-Invariant)  SystemSampleTime=-1  VariantActivationTime=update diagram  AllowFlexibleInterface=on  Latency=0  AutoFrameSizeCalculation=off
      settings: SourceProductName=Simplus Grid Tool
  theta : Outport
  wires:
  Math Function3/1 -> theta/1, [thetax2]  "theta"
  Discrete-Time Integrator1/1 -> Sum/2, Add/2  "theta"
  Constant1/1 -> Math Function1/2
  Transfer Fcn/1 -> PI/1(e)
  Math Function1/1 -> [thetax]  "theta"
  Sum/1 -> Math Function3/1
  Transfer Fcn1/1 -> Scope1/2, Discrete-Time Integrator1/1
  Constant3/1 -> Math Function3/2
  [thetax] -> "abc -> dq (Power-Invariant)5"/2
  Demux6/2 -> Transfer Fcn/1
  PI/1(Out) -> Transfer Fcn1/1, Scope1/1, Discrete-Time Integrator/1  "freq"
  "abc -> dq (Power-Invariant)5"/1 -> Demux6/1
  Add/1 -> 2nd_lpf5/1
  Demux6/1 -> Terminator/1  "vd"
  Vabc/1 -> "abc -> dq (Power-Invariant)5"/1
  Discrete-Time Integrator/1 -> Add/1, Math Function1/1
  [thetax] -> Scope/1
  [thetax2] -> Scope/2
  2nd_lpf5/1 -> Sum/1

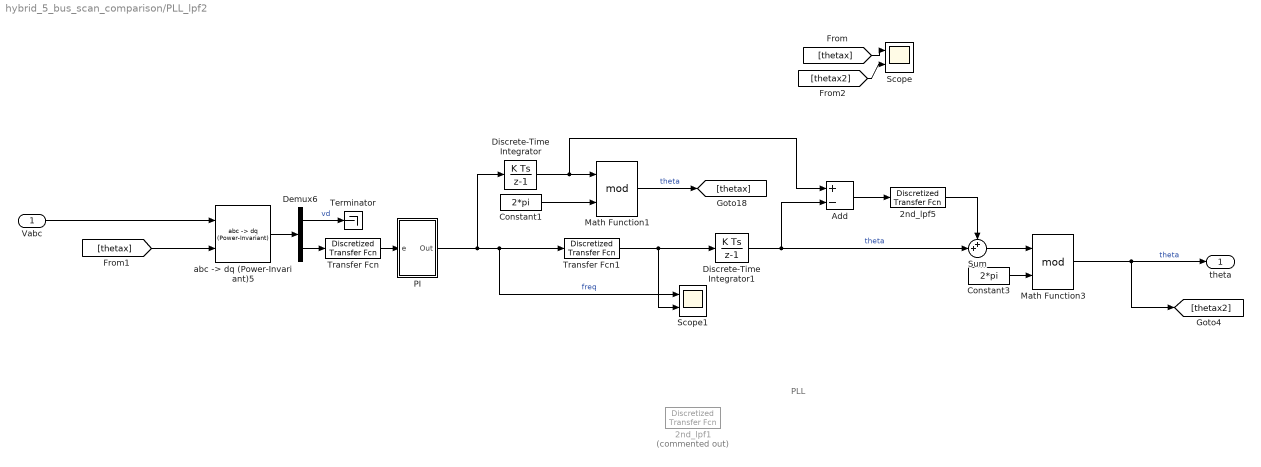
== system hybrid_5_bus_scan_comparison/PLL_lpf2 ==
  note: PLL
  Vabc : Inport
  2nd_lpf1 : discretizing/Discretized Transfer Fcn  Commented=on  Numerator=[wc_lpf^2]  Denominator="[1, 2*k_lpf*wc_lpf,  wc_lpf^2]"  AbsTol=auto  SampleTime=10e-6  method=zoh  Wc=0
  2nd_lpf5 : discretizing/Discretized Transfer Fcn  Numerator=[wc_lpf^2]  Denominator="[1, 2*k_lpf*wc_lpf,  wc_lpf^2]"  AbsTol=auto  SampleTime=50e-6  method=zoh  Wc=0
  Add : Sum  Inputs=+-
  Constant1 : Constant  Value=2*pi
  Constant3 : Constant  Value=2*pi
  Demux6 : Demux  Outputs=2
  Discrete-Time Integrator : DiscreteIntegrator  SampleTime=Ts  ICPrevOutput=DiscIntNeverNeededParam  ICPrevScaledInput=DiscIntNeverNeededParam
  Discrete-Time Integrator1 : DiscreteIntegrator  SampleTime=Ts  ICPrevOutput=DiscIntNeverNeededParam  ICPrevScaledInput=DiscIntNeverNeededParam
  Math Function1 : Math  Operator=mod  SignedPower=on
  Math Function3 : Math  Operator=mod  SignedPower=on
  PI : Subsystem  mask{Kp_PLL=2*pi*fpll, Ki_PLL=(2*pi*fpll)^2/4, IntSat_PLL=20000}
      mask prompts: Kp_PLL "Proportional (P)"; Ki_PLL "Integral (I)"; IntSat_PLL "Integrator Saturation Limit"
      mask DialogControl DescGroupVar Prompt: PLL Parameters
  Scope : Scope  NumInputPorts=2
  Scope1 : Scope  NumInputPorts=2
  Sum : Sum  Inputs=++|
  Terminator : Terminator
  Transfer Fcn : discretizing/Discretized Transfer Fcn  Numerator=[1]  Denominator=[1/(2*pi*50) 1]  AbsTol=auto  SampleTime=50e-6  method=zoh  Wc=0
  Transfer Fcn1 : discretizing/Discretized Transfer Fcn  Numerator=[1]  Denominator=[1/(2*pi*1) 1]  AbsTol=auto  SampleTime=50e-6  method=zoh  Wc=0
  "abc -> dq (Power-Invariant)5" : SimplusGT/abc -> dq (Power-Invariant)  SystemSampleTime=-1  VariantActivationTime=update diagram  AllowFlexibleInterface=on  Latency=0  AutoFrameSizeCalculation=off
      settings: SourceProductName=Simplus Grid Tool
  theta : Outport
  wires:
  Math Function3/1 -> theta/1, [thetax2]  "theta"
  Discrete-Time Integrator1/1 -> Sum/2, Add/2  "theta"
  Constant1/1 -> Math Function1/2
  Transfer Fcn/1 -> PI/1(e)
  Math Function1/1 -> [thetax]  "theta"
  Sum/1 -> Math Function3/1
  Transfer Fcn1/1 -> Scope1/2, Discrete-Time Integrator1/1
  Constant3/1 -> Math Function3/2
  [thetax] -> "abc -> dq (Power-Invariant)5"/2
  Demux6/2 -> Transfer Fcn/1
  PI/1(Out) -> Transfer Fcn1/1, Scope1/1, Discrete-Time Integrator/1  "freq"
  "abc -> dq (Power-Invariant)5"/1 -> Demux6/1
  Add/1 -> 2nd_lpf5/1
  Demux6/1 -> Terminator/1  "vd"
  Vabc/1 -> "abc -> dq (Power-Invariant)5"/1
  Discrete-Time Integrator/1 -> Add/1, Math Function1/1
  [thetax] -> Scope/1
  [thetax2] -> Scope/2
  2nd_lpf5/1 -> Sum/1

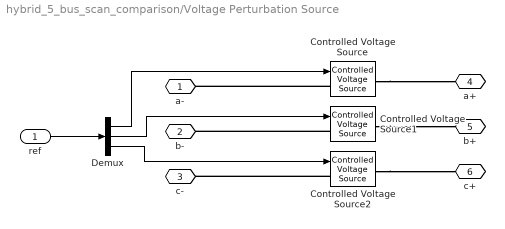
== system hybrid_5_bus_scan_comparison/Voltage Perturbation Source ==
  ref : Inport
  Controlled Voltage Source : spsControlledVoltageSourceLib/Controlled Voltage Source  Initialize=on  Source_Type=AC  Amplitude=0  Phase=0  Frequency=0  Measurements=None
  Controlled Voltage Source1 : spsControlledVoltageSourceLib/Controlled Voltage Source  Initialize=on  Source_Type=AC  Amplitude=0  Phase=0  Frequency=0  Measurements=None
  Controlled Voltage Source2 : spsControlledVoltageSourceLib/Controlled Voltage Source  Initialize=on  Source_Type=AC  Amplitude=0  Phase=0  Frequency=0  Measurements=None
  Demux : Demux  Outputs=3
  a- : PMIOPort  Side=Left
  b- : PMIOPort  Port=2  Side=Left
  c- : PMIOPort  Port=3  Side=Left
  a+ : PMIOPort  Port=4  Side=Right
  b+ : PMIOPort  Port=5  Side=Right
  c+ : PMIOPort  Port=6  Side=Right
  wires:
  Demux/2 -> Controlled Voltage Source1/1
  Demux/3 -> Controlled Voltage Source2/1
  ref/1 -> Demux/1
  Demux/1 -> Controlled Voltage Source/1
  connections:
  Controlled Voltage Source/LConn1 -- a-/RConn1
  Controlled Voltage Source1/RConn1 -- b+/RConn1
  Controlled Voltage Source1/LConn1 -- b-/RConn1
  Controlled Voltage Source/RConn1 -- a+/RConn1
  Controlled Voltage Source2/RConn1 -- c+/RConn1
  Controlled Voltage Source2/LConn1 -- c-/RConn1

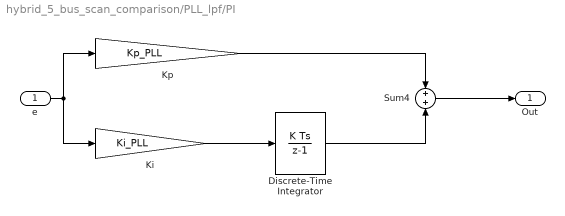
== system hybrid_5_bus_scan_comparison/PLL_lpf/PI ==
  e : Inport
  Discrete-Time Integrator : DiscreteIntegrator  gainval=1  InitialCondition=2*pi*Fbase  SampleTime=Ts  LimitOutput=on  UpperSaturationLimit=2*pi*Fbase + IntSat_PLL  LowerSaturationLimit=2*pi*Fbase - IntSat_PLL  ICPrevOutput=DiscIntNeverNeededParam  ICPrevScaledInput=DiscIntNeverNeededParam
  Ki : Gain  Gain=Ki_PLL  SaturateOnIntegerOverflow=on  OutDataTypeStr=Inherit: Same as input  ParamDataTypeStr=Inherit: Same as input
  Kp : Gain  Gain=Kp_PLL  SaturateOnIntegerOverflow=on  OutDataTypeStr=Inherit: Same as input  ParamDataTypeStr=Inherit: Same as input
  Sum4 : Sum  SaturateOnIntegerOverflow=on
  Out : Outport
  wires:
  Sum4/1 -> Out/1
  Discrete-Time Integrator/1 -> Sum4/2
  e/1 -> Kp/1, Ki/1
  Kp/1 -> Sum4/1
  Ki/1 -> Discrete-Time Integrator/1

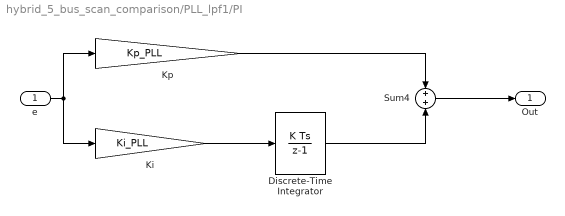
== system hybrid_5_bus_scan_comparison/PLL_lpf1/PI ==
  e : Inport
  Discrete-Time Integrator : DiscreteIntegrator  gainval=1  InitialCondition=2*pi*Fbase  SampleTime=Ts  LimitOutput=on  UpperSaturationLimit=2*pi*Fbase + IntSat_PLL  LowerSaturationLimit=2*pi*Fbase - IntSat_PLL  ICPrevOutput=DiscIntNeverNeededParam  ICPrevScaledInput=DiscIntNeverNeededParam
  Ki : Gain  Gain=Ki_PLL  SaturateOnIntegerOverflow=on  OutDataTypeStr=Inherit: Same as input  ParamDataTypeStr=Inherit: Same as input
  Kp : Gain  Gain=Kp_PLL  SaturateOnIntegerOverflow=on  OutDataTypeStr=Inherit: Same as input  ParamDataTypeStr=Inherit: Same as input
  Sum4 : Sum  SaturateOnIntegerOverflow=on
  Out : Outport
  wires:
  Sum4/1 -> Out/1
  Discrete-Time Integrator/1 -> Sum4/2
  e/1 -> Kp/1, Ki/1
  Kp/1 -> Sum4/1
  Ki/1 -> Discrete-Time Integrator/1

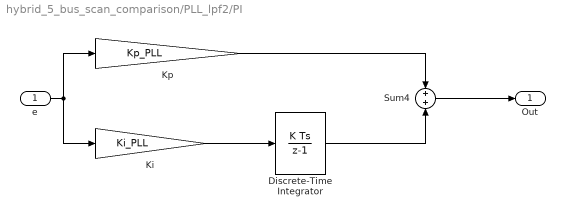
== system hybrid_5_bus_scan_comparison/PLL_lpf2/PI ==
  e : Inport
  Discrete-Time Integrator : DiscreteIntegrator  gainval=1  InitialCondition=2*pi*Fbase  SampleTime=Ts  LimitOutput=on  UpperSaturationLimit=2*pi*Fbase + IntSat_PLL  LowerSaturationLimit=2*pi*Fbase - IntSat_PLL  ICPrevOutput=DiscIntNeverNeededParam  ICPrevScaledInput=DiscIntNeverNeededParam
  Ki : Gain  Gain=Ki_PLL  SaturateOnIntegerOverflow=on  OutDataTypeStr=Inherit: Same as input  ParamDataTypeStr=Inherit: Same as input
  Kp : Gain  Gain=Kp_PLL  SaturateOnIntegerOverflow=on  OutDataTypeStr=Inherit: Same as input  ParamDataTypeStr=Inherit: Same as input
  Sum4 : Sum  SaturateOnIntegerOverflow=on
  Out : Outport
  wires:
  Sum4/1 -> Out/1
  Discrete-Time Integrator/1 -> Sum4/2
  e/1 -> Kp/1, Ki/1
  Kp/1 -> Sum4/1
  Ki/1 -> Discrete-Time Integrator/1

== matlab function hybrid_5_bus_scan_comparison/Frequency_Sweep1/Frequency Sweep ==
  data: EN input; Perturb_DQ output; ResponseDQ input size=[1 2]; FreqSet input; FreqTest input; Cycle input; OutAmp input; Fs input; Interval input; AmpGain input; xD input; FSResult output; FreqPoint output; RecordTrigger output; xD1 output
function [Perturb_DQ, FSResult, FreqPoint, RecordTrigger, xD1] = fcn(EN,ResponseDQ, FreqSet, FreqTest, Cycle, OutAmp, Fs, Interval, AmpGain, xD)
% State variables:
% xD0: case;        xD1:N; total sample points for one period
% xD2:-N;           xD3:n ,sample point count      xD4:k, for cycle count
% xD5: Out_Re       xD6:Out_Im;
% xD7: Sum_Re_d      xD8:Sum_Im_d     xD9:Sum_Re_q     xD10:Sum_Im_q
% xD11, xD12, xD13, xD14----xD7,xD8,xD9,xD10 * dt
% xD15: t, for waiting

% read states
CaseK=xD(1); % case
Ns=xD(2); % total time steps for the set frequency
Nt=xD(3); % total time steps for the tested (calculated) frequency
n=xD(4); % sample point count
kc=xD(5);   % CycleCount
OutD=xD(6); %   Output
OutQ=xD(7);
SumDRe=xD(8); % Integration
SumDIm=xD(9);
SumQRe=xD(10);
SumQIm=xD(11);
FinalDRe=xD(12); % Final Result (complex number)
FinalDIm=xD(13);
FinalQRe=xD(14);
FinalQIm=xD(15);
TWait=xD(16); % wait time

FrequencyNum=length(FreqSet);

if AmpGain==0
    error('gain must not be zero');
end

%% Main Loop
if EN==0   % if Enable 0, reset all variables
    OutD=0;
    OutQ=0;
else
    switch CaseK
        case 0 % the very first round
            kc=1;
            CaseK=1;
        case 1
            if kc>FrequencyNum         %sweep finished. Go to case 9
                OutD=0;
                OutQ=0;   
                CaseK=9; 
            elseif Cycle(kc)==0  % if this frequency is skipped
                kc=kc+1;
            else   
                % prepare to sweep D axis this frequency
                SumDRe=0;
                SumDIm=0;
                SumQRe=0;
                SumQIm=0;
                TWait=0;
                n=0;
                % total time steps for this frequency
                Ns = Fs/FreqSet(kc)*Cycle(kc); % for output count
                Nt = Fs/FreqTest(kc)*Cycle(kc); % for frequency test count
                OutD=OutAmp(kc)*sin(2*pi*Cycle(kc)*n/Ns)*AmpGain;
                OutQ=0;
                n=n+1;
                CaseK=2;
            end
        case 2 % sweep D axis
            OutD=OutAmp(kc)*sin(2*pi*Cycle(kc)*n/Ns)*AmpGain;
        	OutQ=0;
            % D sum
            SumDRe = SumDRe + ResponseDQ(1) * sin(2*pi*Cycle(kc)*(n-1)/Nt);  % Nt is used here, means it is using the tested frequency specified.
            SumDIm = SumDIm + (-1)*ResponseDQ(1) * (-1)*cos(2*pi*Cycle(kc)*(n-1)/Nt);
            % Q sum
            SumQRe = SumQRe + ResponseDQ(2) * sin(2*pi*Cycle(kc)*(n-1)/Nt);
            SumQIm = SumQIm + (-1)*ResponseDQ(2) * (-1)*cos(2*pi*Cycle(kc)*(n-1)/Nt);
            
            if(n<Nt)
                n=n+1;
            else
                OutD=0;
                OutQ=0;
                CaseK=3;
            end
        case 3
            % Set Sweep Results
            FinalDRe = 2*SumDRe*FreqSet(kc)/Cycle(kc)/Fs/OutAmp(kc)/AmpGain;                      
            FinalDIm = 2*SumDIm*FreqSet(kc)/Cycle(kc)/Fs/OutAmp(kc)/AmpGain; 
            FinalQRe = 2*SumQRe*FreqSet(kc)/Cycle(kc)/Fs/OutAmp(kc)/AmpGain;  
            FinalQIm = 2*SumQIm*FreqSet(kc)/Cycle(kc)/Fs/OutAmp(kc)/AmpGain;
            if TWait<Fs*Interval
                TWait=TWait+1;
            else
                TWait=0;
                CaseK=4;
            end
        case 4
            SumDRe=0;
            SumDIm=0;
            SumQRe=0;
            SumQIm=0;
            TWait=0;
            n=0;
            % total time steps for this frequency
            Ns = Fs/FreqSet(kc)*Cycle(kc); % for output count
            Nt = Fs/FreqTest(kc)*Cycle(kc); % for frequency test count
            OutD=0;
            OutQ=OutAmp(kc)*sin(2*pi*Cycle(kc)*n/Ns)*AmpGain;
            n=n+1;
            CaseK=5;
        case 5
            OutD=0;
        	OutQ=OutAmp(kc)*sin(2*pi*Cycle(kc)*n/Ns)*AmpGain;
            % D sum
            SumDRe = SumDRe + ResponseDQ(1) * sin(2*pi*Cycle(kc)*(n-1)/Nt);  % Nt is used here, means it is using the tested frequency specified.
            SumDIm = SumDIm + (-1)*ResponseDQ(1) * (-1)*cos(2*pi*Cycle(kc)*(n-1)/Nt);
            % Q sum
            SumQRe = SumQRe + ResponseDQ(2) * sin(2*pi*Cycle(kc)*(n-1)/Nt);
            SumQIm = SumQIm + (-1)*ResponseDQ(2) * (-1)*cos(2*pi*Cycle(kc)*(n-1)/Nt);
            
            if(n<Nt)
                n=n+1;
            else
                OutD=0;
                OutQ=0;
                CaseK=6;
            end
        case 6
            % Set Sweep Results
            FinalDRe = 2*SumDRe*FreqSet(kc)/Cycle(kc)/Fs/OutAmp(kc)/AmpGain;                      
            FinalDIm = 2*SumDIm*FreqSet(kc)/Cycle(kc)/Fs/OutAmp(kc)/AmpGain; 
            FinalQRe = 2*SumQRe*FreqSet(kc)/Cycle(kc)/Fs/OutAmp(kc)/AmpGain;  
            FinalQIm = 2*SumQIm*FreqSet(kc)/Cycle(kc)/Fs/OutAmp(kc)/AmpGain;
            if TWait<Fs*Interval
                TWait=TWait+1;
            else
                TWait=0;
                kc=kc+1;
                CaseK=1;
            end
        case 9 % nothing
    end
end


%% set outputs
xD1=[CaseK,Ns,Nt,n,kc,OutD,OutQ,SumDRe,SumDIm,SumQRe,SumQIm,FinalDRe,FinalDIm,FinalQRe,FinalQIm,TWait]; % write states
Perturb_DQ=[OutD,OutQ];
1i;
if kc>0 && EN==1
    FSResult = [FinalDRe+FinalDIm*1i, FinalQRe+FinalQIm*1i]; % complex number output
    if kc>FrequencyNum
        kc=FrequencyNum;
    end
    FreqPoint = FreqSet(kc);
    % if TWait>=Fs*Interval/4 && TWait<Fs*Interval*3/4
    %     RecordTrigger=1;
    % else
    %     RecordTrigger=0;
    % end
else
    FSResult=[0,0];
    %RecordTrigger=0;
    FreqPoint=0;
end
if CaseK==3 || CaseK==6
    RecordTrigger=1; % trigger is deleyed for two cycles outside the block.
else
    RecordTrigger=0;
end

end
